simulink model "ZRD_laengs_Simulator_einfach"  (R2021a)
settings: Solver=VariableStepAuto  StartTime=0.0  StopTime=10.0  RelTol=1e-3
values from neighbouring files (symbols this model uses):
  A1 = [-0.4731865809 -87.6450530495 -6.26938451561 0.429096415729 0.00219470810491 -58.2128494877 -0.00953614403282 0.0912875702238 -0.000763325096957 1.66437872449 -0.0741111475602 0.000865723105751 ... (16 elements, 4x4)]    [AB.mat]    (also in ZRD_laengsbewegung.m = A)
  B1 = [-0.0634198470314  -0.0226287671387; -97.6955223213  -53.7881728478; -0.351042475926  5.47598911329; 0.109518795981  -0.0880572116744]    [AB.mat]    (also in ZRD_laengsbewegung.m = B)
  x0 = [a0 0 V0 0]    [ZRD_laengs.m]    (also in ZRD_laengsbewegung.m = [x1filt(1);x2filt(1);x3filt(1);x4filt(1)])
settings Model: Creator=Florian  LastModifiedBy=Fabrizio
settings SolverCC: AlgebraicLoopSolver=TrustRegion
settings DebuggingCC: SFMachineParentedDataDiag=warning

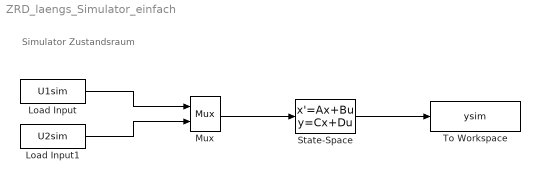
== system ZRD_laengs_Simulator_einfach ==
  note: Simulator Zustandsraum
  Load Input : FromWorkspace  VariableName=U1sim  SampleTime=-1
  Load Input1 : FromWorkspace  VariableName=U2sim  SampleTime=-1
  Mux : Mux  Inputs=2
  State-Space : StateSpace  A=A1  B=B1  C=eye(4,4);  D=zeros(4,2)  InitialCondition=x0
  To Workspace : ToWorkspace  VariableName=ysim  SampleTime=-1
  wires:
  Mux/1 -> State-Space/1
  State-Space/1 -> To Workspace/1
  Load Input/1 -> Mux/1
  Load Input1/1 -> Mux/2
